simulink model "MIMO_FIXED"  (R2017a)
settings: Solver=VariableStepAuto  StartTime=0.0  StopTime=1000  RelTol=1e-3
libraries: dspsigops x80, commchan3 x4, commdigbbndpm3 x2, commfilt2 x2, commsink2 x1, commutil2 x1
(part 5 of 6)

== system MIMO_FIXED/Transceiver7/Interpolation 2/E4 ==
  In1 : Inport
  Data Type Conversion1 : DataTypeConversion  OutDataTypeStr=fixdt(1,18,0)  SaturateOnIntegerOverflow=on
  Data Type Conversion12 : DataTypeConversion  OutDataTypeStr=fixdt(1,11,0)  SaturateOnIntegerOverflow=on
  Data Type Conversion2 : DataTypeConversion  OutDataTypeStr=fixdt(1,19,0)  SaturateOnIntegerOverflow=on
  Data Type Conversion3 : DataTypeConversion  OutDataTypeStr=fixdt(1,16,0)  SaturateOnIntegerOverflow=on
  Data Type Conversion4 : DataTypeConversion  OutDataTypeStr=fixdt(1,18,0)  SaturateOnIntegerOverflow=on
  Data Type Conversion5 : DataTypeConversion  OutDataTypeStr=fixdt(1,19,0)  SaturateOnIntegerOverflow=on
  Delay3 : Delay  DelayLength=1
  Delay4 : Delay  DelayLength=1
  Delay5 : Delay  DelayLength=1
  Gain : Gain
  Gain1 : Gain  Gain=161
  Gain2 : Gain  Gain=315
  Gain3 : Gain  Gain=35
  Sum : Sum
  Sum1 : Sum
  Sum2 : Sum
  Out1 : Outport
  wires:
  Sum1/1 -> Data Type Conversion5/1
  Sum/1 -> Data Type Conversion4/1
  Gain1/1 -> Data Type Conversion1/1
  Delay3/1 -> Sum/2
  Delay4/1 -> Sum1/2
  Gain3/1 -> Data Type Conversion3/1
  Delay5/1 -> Sum2/2
  Gain/1 -> Data Type Conversion12/1
  Data Type Conversion12/1 -> Delay3/1
  Data Type Conversion1/1 -> Sum/1
  Gain2/1 -> Data Type Conversion2/1
  Data Type Conversion2/1 -> Sum1/1
  Data Type Conversion3/1 -> Sum2/1
  Data Type Conversion4/1 -> Delay4/1
  Data Type Conversion5/1 -> Delay5/1
  In1/1 -> Gain2/1, Gain3/1, Gain1/1, Gain/1
  Sum2/1 -> Out1/1

== system MIMO_FIXED/Transceiver7/Interpolation 2/E5 ==
  In1 : Inport
  Data Type Conversion1 : DataTypeConversion  OutDataTypeStr=fixdt(1,19,0)  SaturateOnIntegerOverflow=on
  Data Type Conversion12 : DataTypeConversion  OutDataTypeStr=fixdt(1,18,0)  SaturateOnIntegerOverflow=on
  Data Type Conversion2 : DataTypeConversion  OutDataTypeStr=fixdt(1,17,0)  SaturateOnIntegerOverflow=on
  Data Type Conversion3 : DataTypeConversion  OutDataTypeStr=fixdt(1,19,0)  SaturateOnIntegerOverflow=on
  Delay6 : Delay  DelayLength=1
  Delay7 : Delay  DelayLength=1
  Gain4 : Gain  Gain=120
  Gain5 : Gain  Gain=336
  Gain6 : Gain  Gain=56
  Sum4 : Sum
  Sum5 : Sum
  Out1 : Outport
  wires:
  Gain4/1 -> Data Type Conversion12/1
  Sum4/1 -> Data Type Conversion3/1
  Delay7/1 -> Sum5/2
  Gain6/1 -> Data Type Conversion2/1
  Delay6/1 -> Sum4/2
  Data Type Conversion12/1 -> Delay6/1
  Gain5/1 -> Data Type Conversion1/1
  Data Type Conversion1/1 -> Sum4/1
  Data Type Conversion2/1 -> Sum5/1
  Data Type Conversion3/1 -> Delay7/1
  In1/1 -> Gain6/1, Gain5/1, Gain4/1
  Sum5/1 -> Out1/1

== system MIMO_FIXED/Transceiver7/Interpolation 2/E6 ==
  In1 : Inport
  Data Type Conversion1 : DataTypeConversion  OutDataTypeStr=fixdt(1,20,0)  SaturateOnIntegerOverflow=on
  Data Type Conversion2 : DataTypeConversion  OutDataTypeStr=fixdt(1,20,0)  SaturateOnIntegerOverflow=on
  Data Type Conversion3 : DataTypeConversion  OutDataTypeStr=fixdt(1,17,0)  SaturateOnIntegerOverflow=on
  Delay6 : Delay  DelayLength=1
  Delay7 : Delay  DelayLength=1
  Gain4 : Gain  Gain=84
  Gain5 : Gain  Gain=344
  Sum4 : Sum
  Sum5 : Sum
  Out1 : Outport
  wires:
  Delay7/1 -> Sum5/2
  Gain4/1 -> Data Type Conversion3/1
  Gain5/1 -> Data Type Conversion1/1
  Delay6/1 -> Sum4/2
  Data Type Conversion3/1 -> Sum5/1, Delay6/1
  Data Type Conversion1/1 -> Sum4/1
  Sum4/1 -> Data Type Conversion2/1
  Data Type Conversion2/1 -> Delay7/1
  In1/1 -> Gain5/1, Gain4/1
  Sum5/1 -> Out1/1

== system MIMO_FIXED/Transceiver7/Interpolation 2/E7 ==
  In1 : Inport
  Data Type Conversion1 : DataTypeConversion  OutDataTypeStr=fixdt(1,19,0)  SaturateOnIntegerOverflow=on
  Data Type Conversion12 : DataTypeConversion  OutDataTypeStr=fixdt(1,17,0)  SaturateOnIntegerOverflow=on
  Data Type Conversion2 : DataTypeConversion  OutDataTypeStr=fixdt(1,18,0)  SaturateOnIntegerOverflow=on
  Data Type Conversion3 : DataTypeConversion  OutDataTypeStr=fixdt(1,19,0)  SaturateOnIntegerOverflow=on
  Delay6 : Delay  DelayLength=1
  Delay7 : Delay  DelayLength=1
  Gain4 : Gain  Gain=56
  Gain5 : Gain  Gain=336
  Gain6 : Gain  Gain=120
  Sum4 : Sum
  Sum5 : Sum
  Out1 : Outport
  wires:
  Gain4/1 -> Data Type Conversion12/1
  Sum4/1 -> Data Type Conversion3/1
  Delay7/1 -> Sum5/2
  Gain6/1 -> Data Type Conversion2/1
  Delay6/1 -> Sum4/2
  Data Type Conversion12/1 -> Delay6/1
  Gain5/1 -> Data Type Conversion1/1
  Data Type Conversion1/1 -> Sum4/1
  Data Type Conversion2/1 -> Sum5/1
  Data Type Conversion3/1 -> Delay7/1
  In1/1 -> Gain6/1, Gain5/1, Gain4/1
  Sum5/1 -> Out1/1

== system MIMO_FIXED/Transceiver1/Interpolation 1/Half_band/E0(Z) ==
  Input : Inport
  Data Type Conversion5 : DataTypeConversion  OutDataTypeStr=fixdt(1,23,0)  SaturateOnIntegerOverflow=on
  Delay : Delay  DelayLength=5
  Gain : Gain  Gain=256
  Out1 : Outport
  wires:
  Input/1 -> Gain/1
  Delay/1 -> Out1/1
  Gain/1 -> Data Type Conversion5/1
  Data Type Conversion5/1 -> Delay/1

== system MIMO_FIXED/Transceiver1/Interpolation 1/Half_band/E1(Z) ==
  Input1 : Inport
  10-12 : Gain  Gain=158
  2-20 : Gain
  4-18 : Gain  Gain=-4
  6-16 : Gain  Gain=13
  8-14 : Gain  Gain=-40
  Add{7..10,12..16} (9 alike) : Sum
  Data Type Conversion1 : DataTypeConversion  OutDataTypeStr=fixdt(1,15,0)  SaturateOnIntegerOverflow=on
  Data Type Conversion{10..14} (5 alike) : DataTypeConversion  OutDataTypeStr=fixdt(1,23,0)  SaturateOnIntegerOverflow=on
  Data Type Conversion2 : DataTypeConversion  OutDataTypeStr=fixdt(1,17,0)  SaturateOnIntegerOverflow=on
  Data Type Conversion3 : DataTypeConversion  OutDataTypeStr=fixdt(1,19,0)  SaturateOnIntegerOverflow=on
  Data Type Conversion4 : DataTypeConversion  OutDataTypeStr=fixdt(1,20,0)  SaturateOnIntegerOverflow=on
  Data Type Conversion5 : DataTypeConversion  OutDataTypeStr=fixdt(1,22,0)  SaturateOnIntegerOverflow=on
  Data Type Conversion6 : DataTypeConversion  OutDataTypeStr=fixdt(1,17,0)  SaturateOnIntegerOverflow=on
  Data Type Conversion7 : DataTypeConversion  OutDataTypeStr=fixdt(1,19,0)  SaturateOnIntegerOverflow=on
  Data Type Conversion8 : DataTypeConversion  OutDataTypeStr=fixdt(1,20,0)  SaturateOnIntegerOverflow=on
  Data Type Conversion9 : DataTypeConversion  OutDataTypeStr=fixdt(1,22,0)  SaturateOnIntegerOverflow=on
  Delay{21,23,25,27,29,31,33,35,37} (9 alike) : Delay  DelayLength=1
  Output : Outport
  wires:
  8-14/1 -> Data Type Conversion4/1
  Delay29/1 -> Add12/2  "x[n-11]"
  Add14/1 -> Data Type Conversion12/1
  Input1/1 -> 2-20/1, 10-12/1, 8-14/1, 6-16/1, 4-18/1
  4-18/1 -> Data Type Conversion2/1
  Delay33/1 -> Add14/2
  Add12/1 -> Data Type Conversion10/1
  10-12/1 -> Data Type Conversion5/1
  Delay37/1 -> Add16/2  "x[n-19]"
  6-16/1 -> Data Type Conversion3/1
  Delay25/1 -> Add9/2  "x[n-7]"
  Add7/1 -> Data Type Conversion6/1
  Add15/1 -> Data Type Conversion13/1
  Delay23/1 -> Add8/2  "x[n-5]"
  Delay27/1 -> Add10/2  "x[n-9]"
  Delay31/1 -> Add13/2  "x[n-13]"
  Delay35/1 -> Add15/2  "x[n-17]"
  Delay21/1 -> Add7/2  "x[n-3]"
  2-20/1 -> Data Type Conversion1/1
  Add13/1 -> Data Type Conversion11/1
  Add10/1 -> Data Type Conversion9/1
  Data Type Conversion1/1 -> Delay21/1, Add16/1
  Data Type Conversion2/1 -> Add7/1, Add15/1
  Data Type Conversion3/1 -> Add8/1, Add14/1
  Data Type Conversion4/1 -> Add9/1, Add13/1
  Data Type Conversion5/1 -> Add10/1, Add12/1
  Data Type Conversion6/1 -> Delay23/1
  Add8/1 -> Data Type Conversion7/1
  Data Type Conversion7/1 -> Delay25/1
  Add9/1 -> Data Type Conversion8/1
  Data Type Conversion8/1 -> Delay27/1
  Data Type Conversion9/1 -> Delay29/1
  Data Type Conversion10/1 -> Delay31/1
  Data Type Conversion11/1 -> Delay33/1
  Data Type Conversion12/1 -> Delay35/1
  Data Type Conversion13/1 -> Delay37/1
  Add16/1 -> Data Type Conversion14/1
  Data Type Conversion14/1 -> Output/1

== system MIMO_FIXED/Transceiver1/Interpolation 1/comb_filter/E0 ==
  In1 : Inport
  Data Type Conversion1 : DataTypeConversion  OutDataTypeStr=fixdt(1,19,0)  SaturateOnIntegerOverflow=on
  Data Type Conversion2 : DataTypeConversion  OutDataTypeStr=fixdt(1,18,0)  SaturateOnIntegerOverflow=on
  Data Type Conversion3 : DataTypeConversion  OutDataTypeStr=fixdt(1,11,0)  SaturateOnIntegerOverflow=on
  Data Type Conversion4 : DataTypeConversion  OutDataTypeStr=fixdt(1,20,0)  SaturateOnIntegerOverflow=on
  Data Type Conversion5 : DataTypeConversion  OutDataTypeStr=fixdt(1,20,0)  SaturateOnIntegerOverflow=on
  Data Type Conversion7 : DataTypeConversion  OutDataTypeStr=fixdt(1,16,0)  SaturateOnIntegerOverflow=on
  Delay3 : Delay  DelayLength=1
  Delay4 : Delay  DelayLength=1
  Delay5 : Delay  DelayLength=1
  Gain : Gain  Gain=35
  Gain1 : Gain  Gain=315
  Gain2 : Gain  Gain=161
  Gain3 : Gain
  Sum : Sum
  Sum1 : Sum
  Sum2 : Sum
  Out1 : Outport
  wires:
  Sum1/1 -> Data Type Conversion5/1
  Delay3/1 -> Sum/2
  Delay5/1 -> Sum2/2
  Data Type Conversion7/1 -> Delay3/1
  Gain/1 -> Data Type Conversion7/1
  Gain1/1 -> Data Type Conversion1/1
  Data Type Conversion1/1 -> Sum/1
  Gain2/1 -> Data Type Conversion2/1
  Data Type Conversion3/1 -> Sum2/1
  Gain3/1 -> Data Type Conversion3/1
  Sum/1 -> Data Type Conversion4/1
  Data Type Conversion4/1 -> Delay4/1
  Data Type Conversion2/1 -> Sum1/1
  Delay4/1 -> Sum1/2
  Data Type Conversion5/1 -> Delay5/1
  In1/1 -> Gain2/1, Gain3/1, Gain1/1, Gain/1
  Sum2/1 -> Out1/1

== system MIMO_FIXED/Transceiver1/Interpolation 1/comb_filter/E1 ==
  In1 : Inport
  Data Type Conversion1 : DataTypeConversion  OutDataTypeStr=fixdt(1,19,0)  SaturateOnIntegerOverflow=on
  Data Type Conversion2 : DataTypeConversion  OutDataTypeStr=fixdt(1,19,0)  SaturateOnIntegerOverflow=on
  Data Type Conversion3 : DataTypeConversion  OutDataTypeStr=fixdt(1,13,0)  SaturateOnIntegerOverflow=on
  Data Type Conversion4 : DataTypeConversion  OutDataTypeStr=fixdt(1,19,0)  SaturateOnIntegerOverflow=on
  Data Type Conversion5 : DataTypeConversion  OutDataTypeStr=fixdt(1,20,0)  SaturateOnIntegerOverflow=on
  Data Type Conversion7 : DataTypeConversion  OutDataTypeStr=fixdt(1,15,0)  SaturateOnIntegerOverflow=on
  Delay3 : Delay  DelayLength=1
  Delay4 : Delay  DelayLength=1
  Delay5 : Delay  DelayLength=1
  Gain : Gain  Gain=20
  Gain1 : Gain  Gain=284
  Gain2 : Gain  Gain=204
  Gain3 : Gain  Gain=4
  Sum : Sum
  Sum1 : Sum
  Sum2 : Sum
  Out1 : Outport
  wires:
  Sum/1 -> Data Type Conversion4/1
  Delay3/1 -> Sum/2
  Delay4/1 -> Sum1/2
  Delay5/1 -> Sum2/2
  Gain/1 -> Data Type Conversion7/1
  Data Type Conversion7/1 -> Delay3/1
  Gain1/1 -> Data Type Conversion1/1
  Data Type Conversion1/1 -> Sum/1
  Gain2/1 -> Data Type Conversion2/1
  Data Type Conversion2/1 -> Sum1/1
  Gain3/1 -> Data Type Conversion3/1
  Data Type Conversion3/1 -> Sum2/1
  Data Type Conversion4/1 -> Delay4/1
  Sum1/1 -> Data Type Conversion5/1
  Data Type Conversion5/1 -> Delay5/1
  In1/1 -> Gain2/1, Gain3/1, Gain1/1, Gain/1
  Sum2/1 -> Out1/1

== system MIMO_FIXED/Transceiver1/Interpolation 1/comb_filter/E2 ==
  In1 : Inport
  Data Type Conversion : DataTypeConversion  OutDataTypeStr=fixdt(1,14,0)
  Data Type Conversion1 : DataTypeConversion  OutDataTypeStr=fixdt(1,19,0)
  Data Type Conversion2 : DataTypeConversion  OutDataTypeStr=fixdt(1,19,0)
  Data Type Conversion3 : DataTypeConversion  OutDataTypeStr=fixdt(1,20,0)
  Delay3 : Delay  DelayLength=1
  Delay4 : Delay  DelayLength=1
  Delay5 : Delay  DelayLength=1
  Gain : Gain  Gain=10
  Gain1 : Gain  Gain=246
  Sum : Sum
  Sum1 : Sum
  Sum2 : Sum
  Out1 : Outport
  wires:
  Sum1/1 -> Data Type Conversion3/1
  Delay3/1 -> Sum/2
  Delay4/1 -> Sum1/2
  Delay5/1 -> Sum2/2
  Data Type Conversion/1 -> Delay3/1, Sum2/1
  Gain/1 -> Data Type Conversion/1
  Gain1/1 -> Data Type Conversion1/1
  Data Type Conversion1/1 -> Sum1/1, Sum/1
  Data Type Conversion2/1 -> Delay4/1
  Sum/1 -> Data Type Conversion2/1
  Data Type Conversion3/1 -> Delay5/1
  In1/1 -> Gain1/1, Gain/1
  Sum2/1 -> Out1/1

== system MIMO_FIXED/Transceiver1/Interpolation 1/comb_filter/E3 ==
  In1 : Inport
  Data Type Conversion : DataTypeConversion  OutDataTypeStr=fixdt(1,13,0)
  Data Type Conversion1 : DataTypeConversion  OutDataTypeStr=fixdt(1,19,0)
  Data Type Conversion2 : DataTypeConversion  OutDataTypeStr=fixdt(1,19,0)
  Data Type Conversion3 : DataTypeConversion  OutDataTypeStr=fixdt(1,15,0)
  Data Type Conversion4 : DataTypeConversion  OutDataTypeStr=fixdt(1,19,0)
  Data Type Conversion5 : DataTypeConversion  OutDataTypeStr=fixdt(1,20,0)
  Delay3 : Delay  DelayLength=1
  Delay4 : Delay  DelayLength=1
  Delay5 : Delay  DelayLength=1
  Gain : Gain  Gain=4
  Gain1 : Gain  Gain=204
  Gain2 : Gain  Gain=284
  Gain3 : Gain  Gain=20
  Sum : Sum
  Sum1 : Sum
  Sum2 : Sum
  Out1 : Outport
  wires:
  Delay3/1 -> Sum/2
  Delay4/1 -> Sum1/2
  Delay5/1 -> Sum2/2
  Gain/1 -> Data Type Conversion/1
  Data Type Conversion/1 -> Delay3/1
  Gain1/1 -> Data Type Conversion1/1
  Data Type Conversion1/1 -> Sum/1
  Gain2/1 -> Data Type Conversion2/1
  Data Type Conversion2/1 -> Sum1/1
  Gain3/1 -> Data Type Conversion3/1
  Data Type Conversion3/1 -> Sum2/1
  Sum/1 -> Data Type Conversion4/1
  Data Type Conversion4/1 -> Delay4/1
  Sum1/1 -> Data Type Conversion5/1
  Data Type Conversion5/1 -> Delay5/1
  Sum2/1 -> Out1/1
  In1/1 -> Gain3/1, Gain2/1, Gain1/1, Gain/1

== system MIMO_FIXED/Transceiver1/Interpolation 1/comb_filter/E4 ==
  In1 : Inport
  Data Type Conversion1 : DataTypeConversion  OutDataTypeStr=fixdt(1,18,0)  SaturateOnIntegerOverflow=on
  Data Type Conversion12 : DataTypeConversion  OutDataTypeStr=fixdt(1,11,0)  SaturateOnIntegerOverflow=on
  Data Type Conversion2 : DataTypeConversion  OutDataTypeStr=fixdt(1,19,0)  SaturateOnIntegerOverflow=on
  Data Type Conversion3 : DataTypeConversion  OutDataTypeStr=fixdt(1,16,0)  SaturateOnIntegerOverflow=on
  Data Type Conversion4 : DataTypeConversion  OutDataTypeStr=fixdt(1,18,0)  SaturateOnIntegerOverflow=on
  Data Type Conversion5 : DataTypeConversion  OutDataTypeStr=fixdt(1,19,0)  SaturateOnIntegerOverflow=on
  Delay3 : Delay  DelayLength=1
  Delay4 : Delay  DelayLength=1
  Delay5 : Delay  DelayLength=1
  Gain : Gain
  Gain1 : Gain  Gain=161
  Gain2 : Gain  Gain=315
  Gain3 : Gain  Gain=35
  Sum : Sum
  Sum1 : Sum
  Sum2 : Sum
  Out1 : Outport
  wires:
  Sum1/1 -> Data Type Conversion5/1
  Sum/1 -> Data Type Conversion4/1
  Gain1/1 -> Data Type Conversion1/1
  Delay3/1 -> Sum/2
  Delay4/1 -> Sum1/2
  Gain3/1 -> Data Type Conversion3/1
  Delay5/1 -> Sum2/2
  Gain/1 -> Data Type Conversion12/1
  Data Type Conversion12/1 -> Delay3/1
  Data Type Conversion1/1 -> Sum/1
  Gain2/1 -> Data Type Conversion2/1
  Data Type Conversion2/1 -> Sum1/1
  Data Type Conversion3/1 -> Sum2/1
  Data Type Conversion4/1 -> Delay4/1
  Data Type Conversion5/1 -> Delay5/1
  In1/1 -> Gain2/1, Gain3/1, Gain1/1, Gain/1
  Sum2/1 -> Out1/1

== system MIMO_FIXED/Transceiver1/Interpolation 1/comb_filter/E5 ==
  In1 : Inport
  Data Type Conversion1 : DataTypeConversion  OutDataTypeStr=fixdt(1,19,0)  SaturateOnIntegerOverflow=on
  Data Type Conversion12 : DataTypeConversion  OutDataTypeStr=fixdt(1,18,0)  SaturateOnIntegerOverflow=on
  Data Type Conversion2 : DataTypeConversion  OutDataTypeStr=fixdt(1,17,0)  SaturateOnIntegerOverflow=on
  Data Type Conversion3 : DataTypeConversion  OutDataTypeStr=fixdt(1,19,0)  SaturateOnIntegerOverflow=on
  Delay6 : Delay  DelayLength=1
  Delay7 : Delay  DelayLength=1
  Gain4 : Gain  Gain=120
  Gain5 : Gain  Gain=336
  Gain6 : Gain  Gain=56
  Sum4 : Sum
  Sum5 : Sum
  Out1 : Outport
  wires:
  Gain4/1 -> Data Type Conversion12/1
  Sum4/1 -> Data Type Conversion3/1
  Delay7/1 -> Sum5/2
  Gain6/1 -> Data Type Conversion2/1
  Delay6/1 -> Sum4/2
  Data Type Conversion12/1 -> Delay6/1
  Gain5/1 -> Data Type Conversion1/1
  Data Type Conversion1/1 -> Sum4/1
  Data Type Conversion2/1 -> Sum5/1
  Data Type Conversion3/1 -> Delay7/1
  In1/1 -> Gain6/1, Gain5/1, Gain4/1
  Sum5/1 -> Out1/1

== system MIMO_FIXED/Transceiver1/Interpolation 1/comb_filter/E6 ==
  In1 : Inport
  Data Type Conversion1 : DataTypeConversion  OutDataTypeStr=fixdt(1,20,0)  SaturateOnIntegerOverflow=on
  Data Type Conversion2 : DataTypeConversion  OutDataTypeStr=fixdt(1,20,0)  SaturateOnIntegerOverflow=on
  Data Type Conversion3 : DataTypeConversion  OutDataTypeStr=fixdt(1,17,0)  SaturateOnIntegerOverflow=on
  Delay6 : Delay  DelayLength=1
  Delay7 : Delay  DelayLength=1
  Gain4 : Gain  Gain=84
  Gain5 : Gain  Gain=344
  Sum4 : Sum
  Sum5 : Sum
  Out1 : Outport
  wires:
  Delay7/1 -> Sum5/2
  Gain4/1 -> Data Type Conversion3/1
  Gain5/1 -> Data Type Conversion1/1
  Delay6/1 -> Sum4/2
  Data Type Conversion3/1 -> Sum5/1, Delay6/1
  Data Type Conversion1/1 -> Sum4/1
  Sum4/1 -> Data Type Conversion2/1
  Data Type Conversion2/1 -> Delay7/1
  In1/1 -> Gain5/1, Gain4/1
  Sum5/1 -> Out1/1

== system MIMO_FIXED/Transceiver1/Interpolation 1/comb_filter/E7 ==
  In1 : Inport
  Data Type Conversion1 : DataTypeConversion  OutDataTypeStr=fixdt(1,19,0)  SaturateOnIntegerOverflow=on
  Data Type Conversion12 : DataTypeConversion  OutDataTypeStr=fixdt(1,17,0)  SaturateOnIntegerOverflow=on
  Data Type Conversion2 : DataTypeConversion  OutDataTypeStr=fixdt(1,18,0)  SaturateOnIntegerOverflow=on
  Data Type Conversion3 : DataTypeConversion  OutDataTypeStr=fixdt(1,19,0)  SaturateOnIntegerOverflow=on
  Delay6 : Delay  DelayLength=1
  Delay7 : Delay  DelayLength=1
  Gain4 : Gain  Gain=56
  Gain5 : Gain  Gain=336
  Gain6 : Gain  Gain=120
  Sum4 : Sum
  Sum5 : Sum
  Out1 : Outport
  wires:
  Gain4/1 -> Data Type Conversion12/1
  Sum4/1 -> Data Type Conversion3/1
  Delay7/1 -> Sum5/2
  Gain6/1 -> Data Type Conversion2/1
  Delay6/1 -> Sum4/2
  Data Type Conversion12/1 -> Delay6/1
  Gain5/1 -> Data Type Conversion1/1
  Data Type Conversion1/1 -> Sum4/1
  Data Type Conversion2/1 -> Sum5/1
  Data Type Conversion3/1 -> Delay7/1
  In1/1 -> Gain6/1, Gain5/1, Gain4/1
  Sum5/1 -> Out1/1

== system MIMO_FIXED/Transceiver5/Interpolation 1/Half_band/E0(Z) ==
  Input : Inport
  Data Type Conversion5 : DataTypeConversion  OutDataTypeStr=fixdt(1,23,0)  SaturateOnIntegerOverflow=on
  Delay : Delay  DelayLength=5
  Gain : Gain  Gain=256
  Out1 : Outport
  wires:
  Input/1 -> Gain/1
  Delay/1 -> Out1/1
  Gain/1 -> Data Type Conversion5/1
  Data Type Conversion5/1 -> Delay/1

== system MIMO_FIXED/Transceiver5/Interpolation 1/Half_band/E1(Z) ==
  Input1 : Inport
  10-12 : Gain  Gain=158
  2-20 : Gain
  4-18 : Gain  Gain=-4
  6-16 : Gain  Gain=13
  8-14 : Gain  Gain=-40
  Add{7..10,12..16} (9 alike) : Sum
  Data Type Conversion1 : DataTypeConversion  OutDataTypeStr=fixdt(1,15,0)  SaturateOnIntegerOverflow=on
  Data Type Conversion{10..14} (5 alike) : DataTypeConversion  OutDataTypeStr=fixdt(1,23,0)  SaturateOnIntegerOverflow=on
  Data Type Conversion2 : DataTypeConversion  OutDataTypeStr=fixdt(1,17,0)  SaturateOnIntegerOverflow=on
  Data Type Conversion3 : DataTypeConversion  OutDataTypeStr=fixdt(1,19,0)  SaturateOnIntegerOverflow=on
  Data Type Conversion4 : DataTypeConversion  OutDataTypeStr=fixdt(1,20,0)  SaturateOnIntegerOverflow=on
  Data Type Conversion5 : DataTypeConversion  OutDataTypeStr=fixdt(1,22,0)  SaturateOnIntegerOverflow=on
  Data Type Conversion6 : DataTypeConversion  OutDataTypeStr=fixdt(1,17,0)  SaturateOnIntegerOverflow=on
  Data Type Conversion7 : DataTypeConversion  OutDataTypeStr=fixdt(1,19,0)  SaturateOnIntegerOverflow=on
  Data Type Conversion8 : DataTypeConversion  OutDataTypeStr=fixdt(1,20,0)  SaturateOnIntegerOverflow=on
  Data Type Conversion9 : DataTypeConversion  OutDataTypeStr=fixdt(1,22,0)  SaturateOnIntegerOverflow=on
  Delay{21,23,25,27,29,31,33,35,37} (9 alike) : Delay  DelayLength=1
  Output : Outport
  wires:
  8-14/1 -> Data Type Conversion4/1
  Delay29/1 -> Add12/2  "x[n-11]"
  Add14/1 -> Data Type Conversion12/1
  Input1/1 -> 2-20/1, 10-12/1, 8-14/1, 6-16/1, 4-18/1
  4-18/1 -> Data Type Conversion2/1
  Delay33/1 -> Add14/2
  Add12/1 -> Data Type Conversion10/1
  10-12/1 -> Data Type Conversion5/1
  Delay37/1 -> Add16/2  "x[n-19]"
  6-16/1 -> Data Type Conversion3/1
  Delay25/1 -> Add9/2  "x[n-7]"
  Add7/1 -> Data Type Conversion6/1
  Add15/1 -> Data Type Conversion13/1
  Delay23/1 -> Add8/2  "x[n-5]"
  Delay27/1 -> Add10/2  "x[n-9]"
  Delay31/1 -> Add13/2  "x[n-13]"
  Delay35/1 -> Add15/2  "x[n-17]"
  Delay21/1 -> Add7/2  "x[n-3]"
  2-20/1 -> Data Type Conversion1/1
  Add13/1 -> Data Type Conversion11/1
  Add10/1 -> Data Type Conversion9/1
  Data Type Conversion1/1 -> Delay21/1, Add16/1
  Data Type Conversion2/1 -> Add7/1, Add15/1
  Data Type Conversion3/1 -> Add8/1, Add14/1
  Data Type Conversion4/1 -> Add9/1, Add13/1
  Data Type Conversion5/1 -> Add10/1, Add12/1
  Data Type Conversion6/1 -> Delay23/1
  Add8/1 -> Data Type Conversion7/1
  Data Type Conversion7/1 -> Delay25/1
  Add9/1 -> Data Type Conversion8/1
  Data Type Conversion8/1 -> Delay27/1
  Data Type Conversion9/1 -> Delay29/1
  Data Type Conversion10/1 -> Delay31/1
  Data Type Conversion11/1 -> Delay33/1
  Data Type Conversion12/1 -> Delay35/1
  Data Type Conversion13/1 -> Delay37/1
  Add16/1 -> Data Type Conversion14/1
  Data Type Conversion14/1 -> Output/1

== system MIMO_FIXED/Transceiver5/Interpolation 1/comb_filter/E0 ==
  In1 : Inport
  Data Type Conversion1 : DataTypeConversion  OutDataTypeStr=fixdt(1,19,0)  SaturateOnIntegerOverflow=on
  Data Type Conversion2 : DataTypeConversion  OutDataTypeStr=fixdt(1,18,0)  SaturateOnIntegerOverflow=on
  Data Type Conversion3 : DataTypeConversion  OutDataTypeStr=fixdt(1,11,0)  SaturateOnIntegerOverflow=on
  Data Type Conversion4 : DataTypeConversion  OutDataTypeStr=fixdt(1,20,0)  SaturateOnIntegerOverflow=on
  Data Type Conversion5 : DataTypeConversion  OutDataTypeStr=fixdt(1,20,0)  SaturateOnIntegerOverflow=on
  Data Type Conversion7 : DataTypeConversion  OutDataTypeStr=fixdt(1,16,0)  SaturateOnIntegerOverflow=on
  Delay3 : Delay  DelayLength=1
  Delay4 : Delay  DelayLength=1
  Delay5 : Delay  DelayLength=1
  Gain : Gain  Gain=35
  Gain1 : Gain  Gain=315
  Gain2 : Gain  Gain=161
  Gain3 : Gain
  Sum : Sum
  Sum1 : Sum
  Sum2 : Sum
  Out1 : Outport
  wires:
  Sum1/1 -> Data Type Conversion5/1
  Delay3/1 -> Sum/2
  Delay5/1 -> Sum2/2
  Data Type Conversion7/1 -> Delay3/1
  Gain/1 -> Data Type Conversion7/1
  Gain1/1 -> Data Type Conversion1/1
  Data Type Conversion1/1 -> Sum/1
  Gain2/1 -> Data Type Conversion2/1
  Data Type Conversion3/1 -> Sum2/1
  Gain3/1 -> Data Type Conversion3/1
  Sum/1 -> Data Type Conversion4/1
  Data Type Conversion4/1 -> Delay4/1
  Data Type Conversion2/1 -> Sum1/1
  Delay4/1 -> Sum1/2
  Data Type Conversion5/1 -> Delay5/1
  In1/1 -> Gain2/1, Gain3/1, Gain1/1, Gain/1
  Sum2/1 -> Out1/1

== system MIMO_FIXED/Transceiver5/Interpolation 1/comb_filter/E1 ==
  In1 : Inport
  Data Type Conversion1 : DataTypeConversion  OutDataTypeStr=fixdt(1,19,0)  SaturateOnIntegerOverflow=on
  Data Type Conversion2 : DataTypeConversion  OutDataTypeStr=fixdt(1,19,0)  SaturateOnIntegerOverflow=on
  Data Type Conversion3 : DataTypeConversion  OutDataTypeStr=fixdt(1,13,0)  SaturateOnIntegerOverflow=on
  Data Type Conversion4 : DataTypeConversion  OutDataTypeStr=fixdt(1,19,0)  SaturateOnIntegerOverflow=on
  Data Type Conversion5 : DataTypeConversion  OutDataTypeStr=fixdt(1,20,0)  SaturateOnIntegerOverflow=on
  Data Type Conversion7 : DataTypeConversion  OutDataTypeStr=fixdt(1,15,0)  SaturateOnIntegerOverflow=on
  Delay3 : Delay  DelayLength=1
  Delay4 : Delay  DelayLength=1
  Delay5 : Delay  DelayLength=1
  Gain : Gain  Gain=20
  Gain1 : Gain  Gain=284
  Gain2 : Gain  Gain=204
  Gain3 : Gain  Gain=4
  Sum : Sum
  Sum1 : Sum
  Sum2 : Sum
  Out1 : Outport
  wires:
  Sum/1 -> Data Type Conversion4/1
  Delay3/1 -> Sum/2
  Delay4/1 -> Sum1/2
  Delay5/1 -> Sum2/2
  Gain/1 -> Data Type Conversion7/1
  Data Type Conversion7/1 -> Delay3/1
  Gain1/1 -> Data Type Conversion1/1
  Data Type Conversion1/1 -> Sum/1
  Gain2/1 -> Data Type Conversion2/1
  Data Type Conversion2/1 -> Sum1/1
  Gain3/1 -> Data Type Conversion3/1
  Data Type Conversion3/1 -> Sum2/1
  Data Type Conversion4/1 -> Delay4/1
  Sum1/1 -> Data Type Conversion5/1
  Data Type Conversion5/1 -> Delay5/1
  In1/1 -> Gain2/1, Gain3/1, Gain1/1, Gain/1
  Sum2/1 -> Out1/1

== system MIMO_FIXED/Transceiver5/Interpolation 1/comb_filter/E2 ==
  In1 : Inport
  Data Type Conversion : DataTypeConversion  OutDataTypeStr=fixdt(1,14,0)
  Data Type Conversion1 : DataTypeConversion  OutDataTypeStr=fixdt(1,19,0)
  Data Type Conversion2 : DataTypeConversion  OutDataTypeStr=fixdt(1,19,0)
  Data Type Conversion3 : DataTypeConversion  OutDataTypeStr=fixdt(1,20,0)
  Delay3 : Delay  DelayLength=1
  Delay4 : Delay  DelayLength=1
  Delay5 : Delay  DelayLength=1
  Gain : Gain  Gain=10
  Gain1 : Gain  Gain=246
  Sum : Sum
  Sum1 : Sum
  Sum2 : Sum
  Out1 : Outport
  wires:
  Sum1/1 -> Data Type Conversion3/1
  Delay3/1 -> Sum/2
  Delay4/1 -> Sum1/2
  Delay5/1 -> Sum2/2
  Data Type Conversion/1 -> Delay3/1, Sum2/1
  Gain/1 -> Data Type Conversion/1
  Gain1/1 -> Data Type Conversion1/1
  Data Type Conversion1/1 -> Sum1/1, Sum/1
  Data Type Conversion2/1 -> Delay4/1
  Sum/1 -> Data Type Conversion2/1
  Data Type Conversion3/1 -> Delay5/1
  In1/1 -> Gain1/1, Gain/1
  Sum2/1 -> Out1/1

== system MIMO_FIXED/Transceiver5/Interpolation 1/comb_filter/E3 ==
  In1 : Inport
  Data Type Conversion : DataTypeConversion  OutDataTypeStr=fixdt(1,13,0)
  Data Type Conversion1 : DataTypeConversion  OutDataTypeStr=fixdt(1,19,0)
  Data Type Conversion2 : DataTypeConversion  OutDataTypeStr=fixdt(1,19,0)
  Data Type Conversion3 : DataTypeConversion  OutDataTypeStr=fixdt(1,15,0)
  Data Type Conversion4 : DataTypeConversion  OutDataTypeStr=fixdt(1,19,0)
  Data Type Conversion5 : DataTypeConversion  OutDataTypeStr=fixdt(1,20,0)
  Delay3 : Delay  DelayLength=1
  Delay4 : Delay  DelayLength=1
  Delay5 : Delay  DelayLength=1
  Gain : Gain  Gain=4
  Gain1 : Gain  Gain=204
  Gain2 : Gain  Gain=284
  Gain3 : Gain  Gain=20
  Sum : Sum
  Sum1 : Sum
  Sum2 : Sum
  Out1 : Outport
  wires:
  Delay3/1 -> Sum/2
  Delay4/1 -> Sum1/2
  Delay5/1 -> Sum2/2
  Gain/1 -> Data Type Conversion/1
  Data Type Conversion/1 -> Delay3/1
  Gain1/1 -> Data Type Conversion1/1
  Data Type Conversion1/1 -> Sum/1
  Gain2/1 -> Data Type Conversion2/1
  Data Type Conversion2/1 -> Sum1/1
  Gain3/1 -> Data Type Conversion3/1
  Data Type Conversion3/1 -> Sum2/1
  Sum/1 -> Data Type Conversion4/1
  Data Type Conversion4/1 -> Delay4/1
  Sum1/1 -> Data Type Conversion5/1
  Data Type Conversion5/1 -> Delay5/1
  Sum2/1 -> Out1/1
  In1/1 -> Gain3/1, Gain2/1, Gain1/1, Gain/1

== system MIMO_FIXED/Transceiver5/Interpolation 1/comb_filter/E4 ==
  In1 : Inport
  Data Type Conversion1 : DataTypeConversion  OutDataTypeStr=fixdt(1,18,0)  SaturateOnIntegerOverflow=on
  Data Type Conversion12 : DataTypeConversion  OutDataTypeStr=fixdt(1,11,0)  SaturateOnIntegerOverflow=on
  Data Type Conversion2 : DataTypeConversion  OutDataTypeStr=fixdt(1,19,0)  SaturateOnIntegerOverflow=on
  Data Type Conversion3 : DataTypeConversion  OutDataTypeStr=fixdt(1,16,0)  SaturateOnIntegerOverflow=on
  Data Type Conversion4 : DataTypeConversion  OutDataTypeStr=fixdt(1,18,0)  SaturateOnIntegerOverflow=on
  Data Type Conversion5 : DataTypeConversion  OutDataTypeStr=fixdt(1,19,0)  SaturateOnIntegerOverflow=on
  Delay3 : Delay  DelayLength=1
  Delay4 : Delay  DelayLength=1
  Delay5 : Delay  DelayLength=1
  Gain : Gain
  Gain1 : Gain  Gain=161
  Gain2 : Gain  Gain=315
  Gain3 : Gain  Gain=35
  Sum : Sum
  Sum1 : Sum
  Sum2 : Sum
  Out1 : Outport
  wires:
  Sum1/1 -> Data Type Conversion5/1
  Sum/1 -> Data Type Conversion4/1
  Gain1/1 -> Data Type Conversion1/1
  Delay3/1 -> Sum/2
  Delay4/1 -> Sum1/2
  Gain3/1 -> Data Type Conversion3/1
  Delay5/1 -> Sum2/2
  Gain/1 -> Data Type Conversion12/1
  Data Type Conversion12/1 -> Delay3/1
  Data Type Conversion1/1 -> Sum/1
  Gain2/1 -> Data Type Conversion2/1
  Data Type Conversion2/1 -> Sum1/1
  Data Type Conversion3/1 -> Sum2/1
  Data Type Conversion4/1 -> Delay4/1
  Data Type Conversion5/1 -> Delay5/1
  In1/1 -> Gain2/1, Gain3/1, Gain1/1, Gain/1
  Sum2/1 -> Out1/1

== system MIMO_FIXED/Transceiver5/Interpolation 1/comb_filter/E5 ==
  In1 : Inport
  Data Type Conversion1 : DataTypeConversion  OutDataTypeStr=fixdt(1,19,0)  SaturateOnIntegerOverflow=on
  Data Type Conversion12 : DataTypeConversion  OutDataTypeStr=fixdt(1,18,0)  SaturateOnIntegerOverflow=on
  Data Type Conversion2 : DataTypeConversion  OutDataTypeStr=fixdt(1,17,0)  SaturateOnIntegerOverflow=on
  Data Type Conversion3 : DataTypeConversion  OutDataTypeStr=fixdt(1,19,0)  SaturateOnIntegerOverflow=on
  Delay6 : Delay  DelayLength=1
  Delay7 : Delay  DelayLength=1
  Gain4 : Gain  Gain=120
  Gain5 : Gain  Gain=336
  Gain6 : Gain  Gain=56
  Sum4 : Sum
  Sum5 : Sum
  Out1 : Outport
  wires:
  Gain4/1 -> Data Type Conversion12/1
  Sum4/1 -> Data Type Conversion3/1
  Delay7/1 -> Sum5/2
  Gain6/1 -> Data Type Conversion2/1
  Delay6/1 -> Sum4/2
  Data Type Conversion12/1 -> Delay6/1
  Gain5/1 -> Data Type Conversion1/1
  Data Type Conversion1/1 -> Sum4/1
  Data Type Conversion2/1 -> Sum5/1
  Data Type Conversion3/1 -> Delay7/1
  In1/1 -> Gain6/1, Gain5/1, Gain4/1
  Sum5/1 -> Out1/1

== system MIMO_FIXED/Transceiver5/Interpolation 1/comb_filter/E6 ==
  In1 : Inport
  Data Type Conversion1 : DataTypeConversion  OutDataTypeStr=fixdt(1,20,0)  SaturateOnIntegerOverflow=on
  Data Type Conversion2 : DataTypeConversion  OutDataTypeStr=fixdt(1,20,0)  SaturateOnIntegerOverflow=on
  Data Type Conversion3 : DataTypeConversion  OutDataTypeStr=fixdt(1,17,0)  SaturateOnIntegerOverflow=on
  Delay6 : Delay  DelayLength=1
  Delay7 : Delay  DelayLength=1
  Gain4 : Gain  Gain=84
  Gain5 : Gain  Gain=344
  Sum4 : Sum
  Sum5 : Sum
  Out1 : Outport
  wires:
  Delay7/1 -> Sum5/2
  Gain4/1 -> Data Type Conversion3/1
  Gain5/1 -> Data Type Conversion1/1
  Delay6/1 -> Sum4/2
  Data Type Conversion3/1 -> Sum5/1, Delay6/1
  Data Type Conversion1/1 -> Sum4/1
  Sum4/1 -> Data Type Conversion2/1
  Data Type Conversion2/1 -> Delay7/1
  In1/1 -> Gain5/1, Gain4/1
  Sum5/1 -> Out1/1

== system MIMO_FIXED/Transceiver5/Interpolation 1/comb_filter/E7 ==
  In1 : Inport
  Data Type Conversion1 : DataTypeConversion  OutDataTypeStr=fixdt(1,19,0)  SaturateOnIntegerOverflow=on
  Data Type Conversion12 : DataTypeConversion  OutDataTypeStr=fixdt(1,17,0)  SaturateOnIntegerOverflow=on
  Data Type Conversion2 : DataTypeConversion  OutDataTypeStr=fixdt(1,18,0)  SaturateOnIntegerOverflow=on
  Data Type Conversion3 : DataTypeConversion  OutDataTypeStr=fixdt(1,19,0)  SaturateOnIntegerOverflow=on
  Delay6 : Delay  DelayLength=1
  Delay7 : Delay  DelayLength=1
  Gain4 : Gain  Gain=56
  Gain5 : Gain  Gain=336
  Gain6 : Gain  Gain=120
  Sum4 : Sum
  Sum5 : Sum
  Out1 : Outport
  wires:
  Gain4/1 -> Data Type Conversion12/1
  Sum4/1 -> Data Type Conversion3/1
  Delay7/1 -> Sum5/2
  Gain6/1 -> Data Type Conversion2/1
  Delay6/1 -> Sum4/2
  Data Type Conversion12/1 -> Delay6/1
  Gain5/1 -> Data Type Conversion1/1
  Data Type Conversion1/1 -> Sum4/1
  Data Type Conversion2/1 -> Sum5/1
  Data Type Conversion3/1 -> Delay7/1
  In1/1 -> Gain6/1, Gain5/1, Gain4/1
  Sum5/1 -> Out1/1

== system MIMO_FIXED/Transceiver6/Interpolation 1/Half_band/E0(Z) ==
  Input : Inport
  Data Type Conversion5 : DataTypeConversion  OutDataTypeStr=fixdt(1,23,0)  SaturateOnIntegerOverflow=on
  Delay : Delay  DelayLength=5
  Gain : Gain  Gain=256
  Out1 : Outport
  wires:
  Input/1 -> Gain/1
  Delay/1 -> Out1/1
  Gain/1 -> Data Type Conversion5/1
  Data Type Conversion5/1 -> Delay/1

== system MIMO_FIXED/Transceiver6/Interpolation 1/Half_band/E1(Z) ==
  Input1 : Inport
  10-12 : Gain  Gain=158
  2-20 : Gain
  4-18 : Gain  Gain=-4
  6-16 : Gain  Gain=13
  8-14 : Gain  Gain=-40
  Add{7..10,12..16} (9 alike) : Sum
  Data Type Conversion1 : DataTypeConversion  OutDataTypeStr=fixdt(1,15,0)  SaturateOnIntegerOverflow=on
  Data Type Conversion{10..14} (5 alike) : DataTypeConversion  OutDataTypeStr=fixdt(1,23,0)  SaturateOnIntegerOverflow=on
  Data Type Conversion2 : DataTypeConversion  OutDataTypeStr=fixdt(1,17,0)  SaturateOnIntegerOverflow=on
  Data Type Conversion3 : DataTypeConversion  OutDataTypeStr=fixdt(1,19,0)  SaturateOnIntegerOverflow=on
  Data Type Conversion4 : DataTypeConversion  OutDataTypeStr=fixdt(1,20,0)  SaturateOnIntegerOverflow=on
  Data Type Conversion5 : DataTypeConversion  OutDataTypeStr=fixdt(1,22,0)  SaturateOnIntegerOverflow=on
  Data Type Conversion6 : DataTypeConversion  OutDataTypeStr=fixdt(1,17,0)  SaturateOnIntegerOverflow=on
  Data Type Conversion7 : DataTypeConversion  OutDataTypeStr=fixdt(1,19,0)  SaturateOnIntegerOverflow=on
  Data Type Conversion8 : DataTypeConversion  OutDataTypeStr=fixdt(1,20,0)  SaturateOnIntegerOverflow=on
  Data Type Conversion9 : DataTypeConversion  OutDataTypeStr=fixdt(1,22,0)  SaturateOnIntegerOverflow=on
  Delay{21,23,25,27,29,31,33,35,37} (9 alike) : Delay  DelayLength=1
  Output : Outport
  wires:
  8-14/1 -> Data Type Conversion4/1
  Delay29/1 -> Add12/2  "x[n-11]"
  Add14/1 -> Data Type Conversion12/1
  Input1/1 -> 2-20/1, 10-12/1, 8-14/1, 6-16/1, 4-18/1
  4-18/1 -> Data Type Conversion2/1
  Delay33/1 -> Add14/2
  Add12/1 -> Data Type Conversion10/1
  10-12/1 -> Data Type Conversion5/1
  Delay37/1 -> Add16/2  "x[n-19]"
  6-16/1 -> Data Type Conversion3/1
  Delay25/1 -> Add9/2  "x[n-7]"
  Add7/1 -> Data Type Conversion6/1
  Add15/1 -> Data Type Conversion13/1
  Delay23/1 -> Add8/2  "x[n-5]"
  Delay27/1 -> Add10/2  "x[n-9]"
  Delay31/1 -> Add13/2  "x[n-13]"
  Delay35/1 -> Add15/2  "x[n-17]"
  Delay21/1 -> Add7/2  "x[n-3]"
  2-20/1 -> Data Type Conversion1/1
  Add13/1 -> Data Type Conversion11/1
  Add10/1 -> Data Type Conversion9/1
  Data Type Conversion1/1 -> Delay21/1, Add16/1
  Data Type Conversion2/1 -> Add7/1, Add15/1
  Data Type Conversion3/1 -> Add8/1, Add14/1
  Data Type Conversion4/1 -> Add9/1, Add13/1
  Data Type Conversion5/1 -> Add10/1, Add12/1
  Data Type Conversion6/1 -> Delay23/1
  Add8/1 -> Data Type Conversion7/1
  Data Type Conversion7/1 -> Delay25/1
  Add9/1 -> Data Type Conversion8/1
  Data Type Conversion8/1 -> Delay27/1
  Data Type Conversion9/1 -> Delay29/1
  Data Type Conversion10/1 -> Delay31/1
  Data Type Conversion11/1 -> Delay33/1
  Data Type Conversion12/1 -> Delay35/1
  Data Type Conversion13/1 -> Delay37/1
  Add16/1 -> Data Type Conversion14/1
  Data Type Conversion14/1 -> Output/1

== system MIMO_FIXED/Transceiver6/Interpolation 1/comb_filter/E0 ==
  In1 : Inport
  Data Type Conversion1 : DataTypeConversion  OutDataTypeStr=fixdt(1,19,0)  SaturateOnIntegerOverflow=on
  Data Type Conversion2 : DataTypeConversion  OutDataTypeStr=fixdt(1,18,0)  SaturateOnIntegerOverflow=on
  Data Type Conversion3 : DataTypeConversion  OutDataTypeStr=fixdt(1,11,0)  SaturateOnIntegerOverflow=on
  Data Type Conversion4 : DataTypeConversion  OutDataTypeStr=fixdt(1,20,0)  SaturateOnIntegerOverflow=on
  Data Type Conversion5 : DataTypeConversion  OutDataTypeStr=fixdt(1,20,0)  SaturateOnIntegerOverflow=on
  Data Type Conversion7 : DataTypeConversion  OutDataTypeStr=fixdt(1,16,0)  SaturateOnIntegerOverflow=on
  Delay3 : Delay  DelayLength=1
  Delay4 : Delay  DelayLength=1
  Delay5 : Delay  DelayLength=1
  Gain : Gain  Gain=35
  Gain1 : Gain  Gain=315
  Gain2 : Gain  Gain=161
  Gain3 : Gain
  Sum : Sum
  Sum1 : Sum
  Sum2 : Sum
  Out1 : Outport
  wires:
  Sum1/1 -> Data Type Conversion5/1
  Delay3/1 -> Sum/2
  Delay5/1 -> Sum2/2
  Data Type Conversion7/1 -> Delay3/1
  Gain/1 -> Data Type Conversion7/1
  Gain1/1 -> Data Type Conversion1/1
  Data Type Conversion1/1 -> Sum/1
  Gain2/1 -> Data Type Conversion2/1
  Data Type Conversion3/1 -> Sum2/1
  Gain3/1 -> Data Type Conversion3/1
  Sum/1 -> Data Type Conversion4/1
  Data Type Conversion4/1 -> Delay4/1
  Data Type Conversion2/1 -> Sum1/1
  Delay4/1 -> Sum1/2
  Data Type Conversion5/1 -> Delay5/1
  In1/1 -> Gain2/1, Gain3/1, Gain1/1, Gain/1
  Sum2/1 -> Out1/1

== system MIMO_FIXED/Transceiver6/Interpolation 1/comb_filter/E1 ==
  In1 : Inport
  Data Type Conversion1 : DataTypeConversion  OutDataTypeStr=fixdt(1,19,0)  SaturateOnIntegerOverflow=on
  Data Type Conversion2 : DataTypeConversion  OutDataTypeStr=fixdt(1,19,0)  SaturateOnIntegerOverflow=on
  Data Type Conversion3 : DataTypeConversion  OutDataTypeStr=fixdt(1,13,0)  SaturateOnIntegerOverflow=on
  Data Type Conversion4 : DataTypeConversion  OutDataTypeStr=fixdt(1,19,0)  SaturateOnIntegerOverflow=on
  Data Type Conversion5 : DataTypeConversion  OutDataTypeStr=fixdt(1,20,0)  SaturateOnIntegerOverflow=on
  Data Type Conversion7 : DataTypeConversion  OutDataTypeStr=fixdt(1,15,0)  SaturateOnIntegerOverflow=on
  Delay3 : Delay  DelayLength=1
  Delay4 : Delay  DelayLength=1
  Delay5 : Delay  DelayLength=1
  Gain : Gain  Gain=20
  Gain1 : Gain  Gain=284
  Gain2 : Gain  Gain=204
  Gain3 : Gain  Gain=4
  Sum : Sum
  Sum1 : Sum
  Sum2 : Sum
  Out1 : Outport
  wires:
  Sum/1 -> Data Type Conversion4/1
  Delay3/1 -> Sum/2
  Delay4/1 -> Sum1/2
  Delay5/1 -> Sum2/2
  Gain/1 -> Data Type Conversion7/1
  Data Type Conversion7/1 -> Delay3/1
  Gain1/1 -> Data Type Conversion1/1
  Data Type Conversion1/1 -> Sum/1
  Gain2/1 -> Data Type Conversion2/1
  Data Type Conversion2/1 -> Sum1/1
  Gain3/1 -> Data Type Conversion3/1
  Data Type Conversion3/1 -> Sum2/1
  Data Type Conversion4/1 -> Delay4/1
  Sum1/1 -> Data Type Conversion5/1
  Data Type Conversion5/1 -> Delay5/1
  In1/1 -> Gain2/1, Gain3/1, Gain1/1, Gain/1
  Sum2/1 -> Out1/1

== system MIMO_FIXED/Transceiver6/Interpolation 1/comb_filter/E2 ==
  In1 : Inport
  Data Type Conversion : DataTypeConversion  OutDataTypeStr=fixdt(1,14,0)
  Data Type Conversion1 : DataTypeConversion  OutDataTypeStr=fixdt(1,19,0)
  Data Type Conversion2 : DataTypeConversion  OutDataTypeStr=fixdt(1,19,0)
  Data Type Conversion3 : DataTypeConversion  OutDataTypeStr=fixdt(1,20,0)
  Delay3 : Delay  DelayLength=1
  Delay4 : Delay  DelayLength=1
  Delay5 : Delay  DelayLength=1
  Gain : Gain  Gain=10
  Gain1 : Gain  Gain=246
  Sum : Sum
  Sum1 : Sum
  Sum2 : Sum
  Out1 : Outport
  wires:
  Sum1/1 -> Data Type Conversion3/1
  Delay3/1 -> Sum/2
  Delay4/1 -> Sum1/2
  Delay5/1 -> Sum2/2
  Data Type Conversion/1 -> Delay3/1, Sum2/1
  Gain/1 -> Data Type Conversion/1
  Gain1/1 -> Data Type Conversion1/1
  Data Type Conversion1/1 -> Sum1/1, Sum/1
  Data Type Conversion2/1 -> Delay4/1
  Sum/1 -> Data Type Conversion2/1
  Data Type Conversion3/1 -> Delay5/1
  In1/1 -> Gain1/1, Gain/1
  Sum2/1 -> Out1/1

== system MIMO_FIXED/Transceiver6/Interpolation 1/comb_filter/E3 ==
  In1 : Inport
  Data Type Conversion : DataTypeConversion  OutDataTypeStr=fixdt(1,13,0)
  Data Type Conversion1 : DataTypeConversion  OutDataTypeStr=fixdt(1,19,0)
  Data Type Conversion2 : DataTypeConversion  OutDataTypeStr=fixdt(1,19,0)
  Data Type Conversion3 : DataTypeConversion  OutDataTypeStr=fixdt(1,15,0)
  Data Type Conversion4 : DataTypeConversion  OutDataTypeStr=fixdt(1,19,0)
  Data Type Conversion5 : DataTypeConversion  OutDataTypeStr=fixdt(1,20,0)
  Delay3 : Delay  DelayLength=1
  Delay4 : Delay  DelayLength=1
  Delay5 : Delay  DelayLength=1
  Gain : Gain  Gain=4
  Gain1 : Gain  Gain=204
  Gain2 : Gain  Gain=284
  Gain3 : Gain  Gain=20
  Sum : Sum
  Sum1 : Sum
  Sum2 : Sum
  Out1 : Outport
  wires:
  Delay3/1 -> Sum/2
  Delay4/1 -> Sum1/2
  Delay5/1 -> Sum2/2
  Gain/1 -> Data Type Conversion/1
  Data Type Conversion/1 -> Delay3/1
  Gain1/1 -> Data Type Conversion1/1
  Data Type Conversion1/1 -> Sum/1
  Gain2/1 -> Data Type Conversion2/1
  Data Type Conversion2/1 -> Sum1/1
  Gain3/1 -> Data Type Conversion3/1
  Data Type Conversion3/1 -> Sum2/1
  Sum/1 -> Data Type Conversion4/1
  Data Type Conversion4/1 -> Delay4/1
  Sum1/1 -> Data Type Conversion5/1
  Data Type Conversion5/1 -> Delay5/1
  Sum2/1 -> Out1/1
  In1/1 -> Gain3/1, Gain2/1, Gain1/1, Gain/1

== system MIMO_FIXED/Transceiver6/Interpolation 1/comb_filter/E4 ==
  In1 : Inport
  Data Type Conversion1 : DataTypeConversion  OutDataTypeStr=fixdt(1,18,0)  SaturateOnIntegerOverflow=on
  Data Type Conversion12 : DataTypeConversion  OutDataTypeStr=fixdt(1,11,0)  SaturateOnIntegerOverflow=on
  Data Type Conversion2 : DataTypeConversion  OutDataTypeStr=fixdt(1,19,0)  SaturateOnIntegerOverflow=on
  Data Type Conversion3 : DataTypeConversion  OutDataTypeStr=fixdt(1,16,0)  SaturateOnIntegerOverflow=on
  Data Type Conversion4 : DataTypeConversion  OutDataTypeStr=fixdt(1,18,0)  SaturateOnIntegerOverflow=on
  Data Type Conversion5 : DataTypeConversion  OutDataTypeStr=fixdt(1,19,0)  SaturateOnIntegerOverflow=on
  Delay3 : Delay  DelayLength=1
  Delay4 : Delay  DelayLength=1
  Delay5 : Delay  DelayLength=1
  Gain : Gain
  Gain1 : Gain  Gain=161
  Gain2 : Gain  Gain=315
  Gain3 : Gain  Gain=35
  Sum : Sum
  Sum1 : Sum
  Sum2 : Sum
  Out1 : Outport
  wires:
  Sum1/1 -> Data Type Conversion5/1
  Sum/1 -> Data Type Conversion4/1
  Gain1/1 -> Data Type Conversion1/1
  Delay3/1 -> Sum/2
  Delay4/1 -> Sum1/2
  Gain3/1 -> Data Type Conversion3/1
  Delay5/1 -> Sum2/2
  Gain/1 -> Data Type Conversion12/1
  Data Type Conversion12/1 -> Delay3/1
  Data Type Conversion1/1 -> Sum/1
  Gain2/1 -> Data Type Conversion2/1
  Data Type Conversion2/1 -> Sum1/1
  Data Type Conversion3/1 -> Sum2/1
  Data Type Conversion4/1 -> Delay4/1
  Data Type Conversion5/1 -> Delay5/1
  In1/1 -> Gain2/1, Gain3/1, Gain1/1, Gain/1
  Sum2/1 -> Out1/1

== system MIMO_FIXED/Transceiver6/Interpolation 1/comb_filter/E5 ==
  In1 : Inport
  Data Type Conversion1 : DataTypeConversion  OutDataTypeStr=fixdt(1,19,0)  SaturateOnIntegerOverflow=on
  Data Type Conversion12 : DataTypeConversion  OutDataTypeStr=fixdt(1,18,0)  SaturateOnIntegerOverflow=on
  Data Type Conversion2 : DataTypeConversion  OutDataTypeStr=fixdt(1,17,0)  SaturateOnIntegerOverflow=on
  Data Type Conversion3 : DataTypeConversion  OutDataTypeStr=fixdt(1,19,0)  SaturateOnIntegerOverflow=on
  Delay6 : Delay  DelayLength=1
  Delay7 : Delay  DelayLength=1
  Gain4 : Gain  Gain=120
  Gain5 : Gain  Gain=336
  Gain6 : Gain  Gain=56
  Sum4 : Sum
  Sum5 : Sum
  Out1 : Outport
  wires:
  Gain4/1 -> Data Type Conversion12/1
  Sum4/1 -> Data Type Conversion3/1
  Delay7/1 -> Sum5/2
  Gain6/1 -> Data Type Conversion2/1
  Delay6/1 -> Sum4/2
  Data Type Conversion12/1 -> Delay6/1
  Gain5/1 -> Data Type Conversion1/1
  Data Type Conversion1/1 -> Sum4/1
  Data Type Conversion2/1 -> Sum5/1
  Data Type Conversion3/1 -> Delay7/1
  In1/1 -> Gain6/1, Gain5/1, Gain4/1
  Sum5/1 -> Out1/1

== system MIMO_FIXED/Transceiver6/Interpolation 1/comb_filter/E6 ==
  In1 : Inport
  Data Type Conversion1 : DataTypeConversion  OutDataTypeStr=fixdt(1,20,0)  SaturateOnIntegerOverflow=on
  Data Type Conversion2 : DataTypeConversion  OutDataTypeStr=fixdt(1,20,0)  SaturateOnIntegerOverflow=on
  Data Type Conversion3 : DataTypeConversion  OutDataTypeStr=fixdt(1,17,0)  SaturateOnIntegerOverflow=on
  Delay6 : Delay  DelayLength=1
  Delay7 : Delay  DelayLength=1
  Gain4 : Gain  Gain=84
  Gain5 : Gain  Gain=344
  Sum4 : Sum
  Sum5 : Sum
  Out1 : Outport
  wires:
  Delay7/1 -> Sum5/2
  Gain4/1 -> Data Type Conversion3/1
  Gain5/1 -> Data Type Conversion1/1
  Delay6/1 -> Sum4/2
  Data Type Conversion3/1 -> Sum5/1, Delay6/1
  Data Type Conversion1/1 -> Sum4/1
  Sum4/1 -> Data Type Conversion2/1
  Data Type Conversion2/1 -> Delay7/1
  In1/1 -> Gain5/1, Gain4/1
  Sum5/1 -> Out1/1

== system MIMO_FIXED/Transceiver6/Interpolation 1/comb_filter/E7 ==
  In1 : Inport
  Data Type Conversion1 : DataTypeConversion  OutDataTypeStr=fixdt(1,19,0)  SaturateOnIntegerOverflow=on
  Data Type Conversion12 : DataTypeConversion  OutDataTypeStr=fixdt(1,17,0)  SaturateOnIntegerOverflow=on
  Data Type Conversion2 : DataTypeConversion  OutDataTypeStr=fixdt(1,18,0)  SaturateOnIntegerOverflow=on
  Data Type Conversion3 : DataTypeConversion  OutDataTypeStr=fixdt(1,19,0)  SaturateOnIntegerOverflow=on
  Delay6 : Delay  DelayLength=1
  Delay7 : Delay  DelayLength=1
  Gain4 : Gain  Gain=56
  Gain5 : Gain  Gain=336
  Gain6 : Gain  Gain=120
  Sum4 : Sum
  Sum5 : Sum
  Out1 : Outport
  wires:
  Gain4/1 -> Data Type Conversion12/1
  Sum4/1 -> Data Type Conversion3/1
  Delay7/1 -> Sum5/2
  Gain6/1 -> Data Type Conversion2/1
  Delay6/1 -> Sum4/2
  Data Type Conversion12/1 -> Delay6/1
  Gain5/1 -> Data Type Conversion1/1
  Data Type Conversion1/1 -> Sum4/1
  Data Type Conversion2/1 -> Sum5/1
  Data Type Conversion3/1 -> Delay7/1
  In1/1 -> Gain6/1, Gain5/1, Gain4/1
  Sum5/1 -> Out1/1

== system MIMO_FIXED/Transceiver7/Interpolation 1/Half_band/E0(Z) ==
  Input : Inport
  Data Type Conversion5 : DataTypeConversion  OutDataTypeStr=fixdt(1,23,0)  SaturateOnIntegerOverflow=on
  Delay : Delay  DelayLength=5
  Gain : Gain  Gain=256
  Out1 : Outport
  wires:
  Input/1 -> Gain/1
  Delay/1 -> Out1/1
  Gain/1 -> Data Type Conversion5/1
  Data Type Conversion5/1 -> Delay/1

== system MIMO_FIXED/Transceiver7/Interpolation 1/Half_band/E1(Z) ==
  Input1 : Inport
  10-12 : Gain  Gain=158
  2-20 : Gain
  4-18 : Gain  Gain=-4
  6-16 : Gain  Gain=13
  8-14 : Gain  Gain=-40
  Add{7..10,12..16} (9 alike) : Sum
  Data Type Conversion1 : DataTypeConversion  OutDataTypeStr=fixdt(1,15,0)  SaturateOnIntegerOverflow=on
  Data Type Conversion{10..14} (5 alike) : DataTypeConversion  OutDataTypeStr=fixdt(1,23,0)  SaturateOnIntegerOverflow=on
  Data Type Conversion2 : DataTypeConversion  OutDataTypeStr=fixdt(1,17,0)  SaturateOnIntegerOverflow=on
  Data Type Conversion3 : DataTypeConversion  OutDataTypeStr=fixdt(1,19,0)  SaturateOnIntegerOverflow=on
  Data Type Conversion4 : DataTypeConversion  OutDataTypeStr=fixdt(1,20,0)  SaturateOnIntegerOverflow=on
  Data Type Conversion5 : DataTypeConversion  OutDataTypeStr=fixdt(1,22,0)  SaturateOnIntegerOverflow=on
  Data Type Conversion6 : DataTypeConversion  OutDataTypeStr=fixdt(1,17,0)  SaturateOnIntegerOverflow=on
  Data Type Conversion7 : DataTypeConversion  OutDataTypeStr=fixdt(1,19,0)  SaturateOnIntegerOverflow=on
  Data Type Conversion8 : DataTypeConversion  OutDataTypeStr=fixdt(1,20,0)  SaturateOnIntegerOverflow=on
  Data Type Conversion9 : DataTypeConversion  OutDataTypeStr=fixdt(1,22,0)  SaturateOnIntegerOverflow=on
  Delay{21,23,25,27,29,31,33,35,37} (9 alike) : Delay  DelayLength=1
  Output : Outport
  wires:
  8-14/1 -> Data Type Conversion4/1
  Delay29/1 -> Add12/2  "x[n-11]"
  Add14/1 -> Data Type Conversion12/1
  Input1/1 -> 2-20/1, 10-12/1, 8-14/1, 6-16/1, 4-18/1
  4-18/1 -> Data Type Conversion2/1
  Delay33/1 -> Add14/2
  Add12/1 -> Data Type Conversion10/1
  10-12/1 -> Data Type Conversion5/1
  Delay37/1 -> Add16/2  "x[n-19]"
  6-16/1 -> Data Type Conversion3/1
  Delay25/1 -> Add9/2  "x[n-7]"
  Add7/1 -> Data Type Conversion6/1
  Add15/1 -> Data Type Conversion13/1
  Delay23/1 -> Add8/2  "x[n-5]"
  Delay27/1 -> Add10/2  "x[n-9]"
  Delay31/1 -> Add13/2  "x[n-13]"
  Delay35/1 -> Add15/2  "x[n-17]"
  Delay21/1 -> Add7/2  "x[n-3]"
  2-20/1 -> Data Type Conversion1/1
  Add13/1 -> Data Type Conversion11/1
  Add10/1 -> Data Type Conversion9/1
  Data Type Conversion1/1 -> Delay21/1, Add16/1
  Data Type Conversion2/1 -> Add7/1, Add15/1
  Data Type Conversion3/1 -> Add8/1, Add14/1
  Data Type Conversion4/1 -> Add9/1, Add13/1
  Data Type Conversion5/1 -> Add10/1, Add12/1
  Data Type Conversion6/1 -> Delay23/1
  Add8/1 -> Data Type Conversion7/1
  Data Type Conversion7/1 -> Delay25/1
  Add9/1 -> Data Type Conversion8/1
  Data Type Conversion8/1 -> Delay27/1
  Data Type Conversion9/1 -> Delay29/1
  Data Type Conversion10/1 -> Delay31/1
  Data Type Conversion11/1 -> Delay33/1
  Data Type Conversion12/1 -> Delay35/1
  Data Type Conversion13/1 -> Delay37/1
  Add16/1 -> Data Type Conversion14/1
  Data Type Conversion14/1 -> Output/1

== system MIMO_FIXED/Transceiver7/Interpolation 1/comb_filter/E0 ==
  In1 : Inport
  Data Type Conversion1 : DataTypeConversion  OutDataTypeStr=fixdt(1,19,0)  SaturateOnIntegerOverflow=on
  Data Type Conversion2 : DataTypeConversion  OutDataTypeStr=fixdt(1,18,0)  SaturateOnIntegerOverflow=on
  Data Type Conversion3 : DataTypeConversion  OutDataTypeStr=fixdt(1,11,0)  SaturateOnIntegerOverflow=on
  Data Type Conversion4 : DataTypeConversion  OutDataTypeStr=fixdt(1,20,0)  SaturateOnIntegerOverflow=on
  Data Type Conversion5 : DataTypeConversion  OutDataTypeStr=fixdt(1,20,0)  SaturateOnIntegerOverflow=on
  Data Type Conversion7 : DataTypeConversion  OutDataTypeStr=fixdt(1,16,0)  SaturateOnIntegerOverflow=on
  Delay3 : Delay  DelayLength=1
  Delay4 : Delay  DelayLength=1
  Delay5 : Delay  DelayLength=1
  Gain : Gain  Gain=35
  Gain1 : Gain  Gain=315
  Gain2 : Gain  Gain=161
  Gain3 : Gain
  Sum : Sum
  Sum1 : Sum
  Sum2 : Sum
  Out1 : Outport
  wires:
  Sum1/1 -> Data Type Conversion5/1
  Delay3/1 -> Sum/2
  Delay5/1 -> Sum2/2
  Data Type Conversion7/1 -> Delay3/1
  Gain/1 -> Data Type Conversion7/1
  Gain1/1 -> Data Type Conversion1/1
  Data Type Conversion1/1 -> Sum/1
  Gain2/1 -> Data Type Conversion2/1
  Data Type Conversion3/1 -> Sum2/1
  Gain3/1 -> Data Type Conversion3/1
  Sum/1 -> Data Type Conversion4/1
  Data Type Conversion4/1 -> Delay4/1
  Data Type Conversion2/1 -> Sum1/1
  Delay4/1 -> Sum1/2
  Data Type Conversion5/1 -> Delay5/1
  In1/1 -> Gain2/1, Gain3/1, Gain1/1, Gain/1
  Sum2/1 -> Out1/1
